simulink model "gm_test_phase_voltages_without_delays"  (R2022a)
settings: Solver=FixedStepDiscrete  StartTime=0.0  StopTime=10.0  RelTol=1e-3
undefined symbols (not defined in the file or in its folder): f_c, u_dc
libraries: hdlmdlgenlib x22, simulink x2
(part 2 of 5)

== system gm_test_phase_voltages_without_delays/Phase_voltages_per_switching_state1/Detect Rise Positive1/Positive ==
  u : Inport  OutDataTypeStr=boolean  SampleTime=1e-08
  Compare : RelationalOperator  Operator=>  OutDataTypeStr=boolean  ZeroCross=off
  Constant : Constant  DisableCoverage=on  Value=0  OutDataTypeStr=Inherit: Inherit via back propagation  SampleTime=-1  PreserveConstantTs=on
  y : Outport  SampleTime=1e-08
  wires:
  Compare/1 -> y/1
  Constant/1 -> Compare/2
  u/1 -> Compare/1

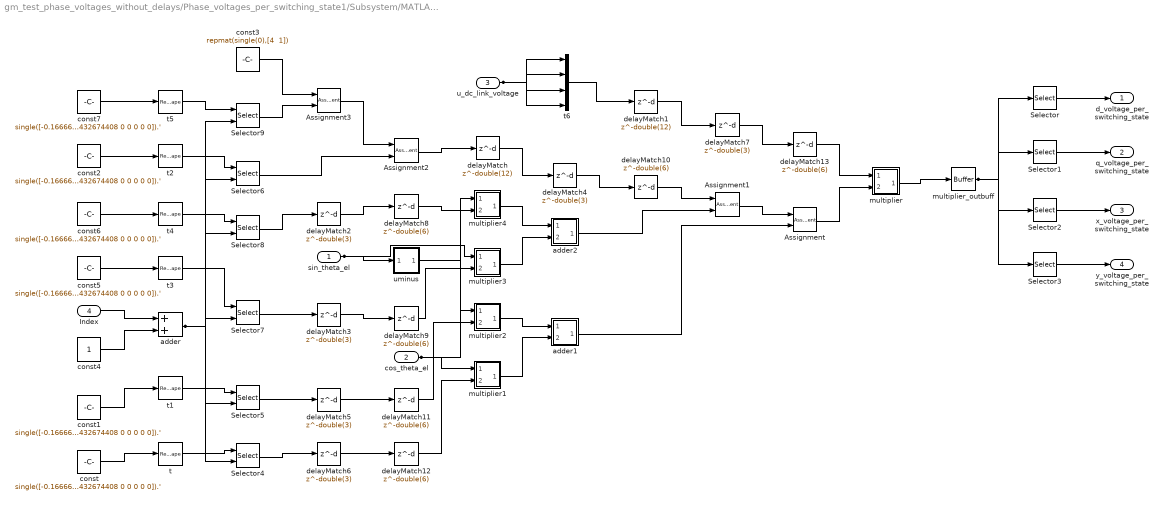
== system gm_test_phase_voltages_without_delays/Phase_voltages_per_switching_state1/Subsystem/MATLAB Function ==
  sin_theta_el : Inport  OutDataTypeStr=single  PortDimensions=1  SampleTime=1e-08
  cos_theta_el : Inport  Port=2  OutDataTypeStr=single  PortDimensions=1  SampleTime=1e-08
  u_dc_link_voltage : Inport  Port=3  OutDataTypeStr=single  PortDimensions=1  SampleTime=1e-08
  Index : Inport  Port=4  OutDataTypeStr=int32  PortDimensions=1  SampleTime=1e-08
  Assignment : Assignment  NumberOfDimensions=2  SampleTime=1e-08  IndexOptions=Index vector (dialog),Index vector (dialog)  Indices=double(2),double(1)  OutputSizes=double(0),double(0)
  Assignment1 : Assignment  NumberOfDimensions=2  SampleTime=1e-08  IndexOptions=Index vector (dialog),Index vector (dialog)  Indices=double(1),double(1)  OutputSizes=double(0),double(0)
  Assignment2 : Assignment  NumberOfDimensions=2  SampleTime=1e-08  IndexOptions=Index vector (dialog),Index vector (dialog)  Indices=double(4),double(1)  OutputSizes=double(0),double(0)
  Assignment3 : Assignment  NumberOfDimensions=2  SampleTime=1e-08  IndexOptions=Index vector (dialog),Index vector (dialog)  Indices=double(3),double(1)  OutputSizes=double(0),double(0)
  Selector : Selector  NumberOfDimensions=2  SampleTime=1e-08  IndexOptions=Index vector (dialog),Index vector (dialog)  Indices=double(1),double(1)  OutputSizes=double(0),double(0)
  Selector1 : Selector  NumberOfDimensions=2  SampleTime=1e-08  IndexOptions=Index vector (dialog),Index vector (dialog)  Indices=double(2),double(1)  OutputSizes=double(0),double(0)
  Selector2 : Selector  NumberOfDimensions=2  SampleTime=1e-08  IndexOptions=Index vector (dialog),Index vector (dialog)  Indices=double(3),double(1)  OutputSizes=double(0),double(0)
  Selector3 : Selector  NumberOfDimensions=2  SampleTime=1e-08  IndexOptions=Index vector (dialog),Index vector (dialog)  Indices=double(4),double(1)  OutputSizes=double(0),double(0)
  Selector4 : Selector  NumberOfDimensions=2  SampleTime=1e-08  IndexOptions=Index vector (dialog),Index vector (port)  Indices=double(2),double(-1)  OutputSizes=double(0),double(0)
  Selector5 : Selector  NumberOfDimensions=2  SampleTime=1e-08  IndexOptions=Index vector (dialog),Index vector (port)  Indices=double(1),double(-1)  OutputSizes=double(0),double(0)
  Selector6 : Selector  NumberOfDimensions=2  SampleTime=1e-08  IndexOptions=Index vector (dialog),Index vector (port)  Indices=double(4),double(-1)  OutputSizes=double(0),double(0)
  Selector7 : Selector  NumberOfDimensions=2  SampleTime=1e-08  IndexOptions=Index vector (dialog),Index vector (port)  Indices=double(2),double(-1)  OutputSizes=double(0),double(0)
  Selector8 : Selector  NumberOfDimensions=2  SampleTime=1e-08  IndexOptions=Index vector (dialog),Index vector (port)  Indices=double(1),double(-1)  OutputSizes=double(0),double(0)
  Selector9 : Selector  NumberOfDimensions=2  SampleTime=1e-08  IndexOptions=Index vector (dialog),Index vector (port)  Indices=double(3),double(-1)  OutputSizes=double(0),double(0)
  adder : Sum  AccumDataTypeStr=int32  OutDataTypeStr=int32  RndMeth=Nearest  SaturateOnIntegerOverflow=on  SampleTime=1e-08
  adder1 : Subsystem
      mask Display: disp('NFP\nadd');
  adder2 : Subsystem
      mask Display: disp('NFP\nadd');
  const{,1..2,5..7} (6 alike) : Constant  Value=single([-0.1666666716337204 -0.28867512941360474 -0.1666666716337204 0.28867512941360474 0.1666666716337204 -0.28867512941360474 0.1666666716337204 0.28867512941360474 -0.3333333432674408 0 -0.3333333432674408 0 0 0 0 0]).'  VectorParams1D=off  OutDataTypeStr=single  SampleTime=1e-08
  const3 : Constant  Value="repmat(single(0),[4  1])"  VectorParams1D=off  OutDataTypeStr=single  SampleTime=1e-08
  const4 : Constant  VectorParams1D=off  OutDataTypeStr=int32  SampleTime=1e-08
  delayMatch : Delay  DelayLength=double(12)  InitialCondition=0  SampleTime=1e-08
  delayMatch1 : Delay  DelayLength=double(12)  InitialCondition=0  SampleTime=1e-08
  delayMatch{8..13} (6 alike) : Delay  DelayLength=double(6)  InitialCondition=0  SampleTime=1e-08
  delayMatch{2..7} (6 alike) : Delay  DelayLength=double(3)  InitialCondition=0  SampleTime=1e-08
  multiplier : Subsystem
      mask Display: disp('NFP\nmul');
  multiplier1 : Subsystem
      mask Display: disp('NFP\nmul');
  multiplier2 : Subsystem
      mask Display: disp('NFP\nmul');
  multiplier3 : Subsystem
      mask Display: disp('NFP\nmul');
  multiplier4 : Subsystem
      mask Display: disp('NFP\nmul');
  multiplier_outbuff : hdlmdlgenlib/Buffer
      settings: SourceProductBaseCode=SL
  t{,1..5} (6 alike) : Reshape  OutputDimensionality=Customize  OutputDimensions=[4,4]
  t6 : Mux
  uminus : Subsystem
      mask Display: disp('NFP\numinus');
  d_voltage_per_switching_state : Outport  SampleTime=1e-08  VectorParamsAs1DForOutWhenUnconnected=off
  q_voltage_per_switching_state : Outport  Port=2  SampleTime=1e-08
  x_voltage_per_switching_state : Outport  Port=3  SampleTime=1e-08
  y_voltage_per_switching_state : Outport  Port=4  SampleTime=1e-08
  wires:
  Selector/1 -> d_voltage_per_switching_state/1
  Selector1/1 -> q_voltage_per_switching_state/1
  Selector2/1 -> x_voltage_per_switching_state/1
  Selector3/1 -> y_voltage_per_switching_state/1
  multiplier_outbuff/1 -> Selector3/1, Selector2/1, Selector1/1, Selector/1
  Assignment/1 -> multiplier/2(In2)
  Assignment1/1 -> Assignment/1
  delayMatch10/1 -> Assignment1/1
  delayMatch12/1 -> multiplier1/2(In2)
  delayMatch11/1 -> multiplier2/2(In2)
  Selector6/1 -> Assignment2/2
  Assignment3/1 -> Assignment2/1
  adder/1 -> Selector9/2, Selector8/2, Selector7/2, Selector6/2, Selector5/2, Selector4/2
  t/1 -> Selector4/1
  t1/1 -> Selector5/1
  delayMatch9/1 -> multiplier3/2(In2)
  delayMatch8/1 -> multiplier4/2(In2)
  t2/1 -> Selector6/1
  Selector9/1 -> Assignment3/2
  const3/1 -> Assignment3/1
  const4/1 -> adder/2
  t3/1 -> Selector7/1
  t4/1 -> Selector8/1
  t5/1 -> Selector9/1
  const/1 -> t/1
  const1/1 -> t1/1
  const2/1 -> t2/1
  const5/1 -> t3/1
  const6/1 -> t4/1
  const7/1 -> t5/1
  delayMatch13/1 -> multiplier/1(In1)
  multiplier/1(Out1) -> multiplier_outbuff/1
  adder1/1(Out1) -> Assignment/2
  multiplier1/1(Out1) -> adder1/2(In2)
  multiplier2/1(Out1) -> adder1/1(In1)
  adder2/1(Out1) -> Assignment1/2
  uminus/1(Out1) -> multiplier2/1(In1)
  multiplier3/1(Out1) -> adder2/2(In2)
  multiplier4/1(Out1) -> adder2/1(In1)
  Assignment2/1 -> delayMatch/1
  t6/1 -> delayMatch1/1
  Selector8/1 -> delayMatch2/1
  Selector7/1 -> delayMatch3/1
  delayMatch/1 -> delayMatch4/1
  Selector5/1 -> delayMatch5/1
  Selector4/1 -> delayMatch6/1
  delayMatch1/1 -> delayMatch7/1
  delayMatch2/1 -> delayMatch8/1
  delayMatch3/1 -> delayMatch9/1
  delayMatch4/1 -> delayMatch10/1
  delayMatch5/1 -> delayMatch11/1
  delayMatch6/1 -> delayMatch12/1
  delayMatch7/1 -> delayMatch13/1
  sin_theta_el/1 -> multiplier3/1(In1), uminus/1(In1)
  cos_theta_el/1 -> multiplier4/1(In1), multiplier1/1(In1)
  u_dc_link_voltage/1 -> t6/4, t6/3, t6/2, t6/1
  Index/1 -> adder/1

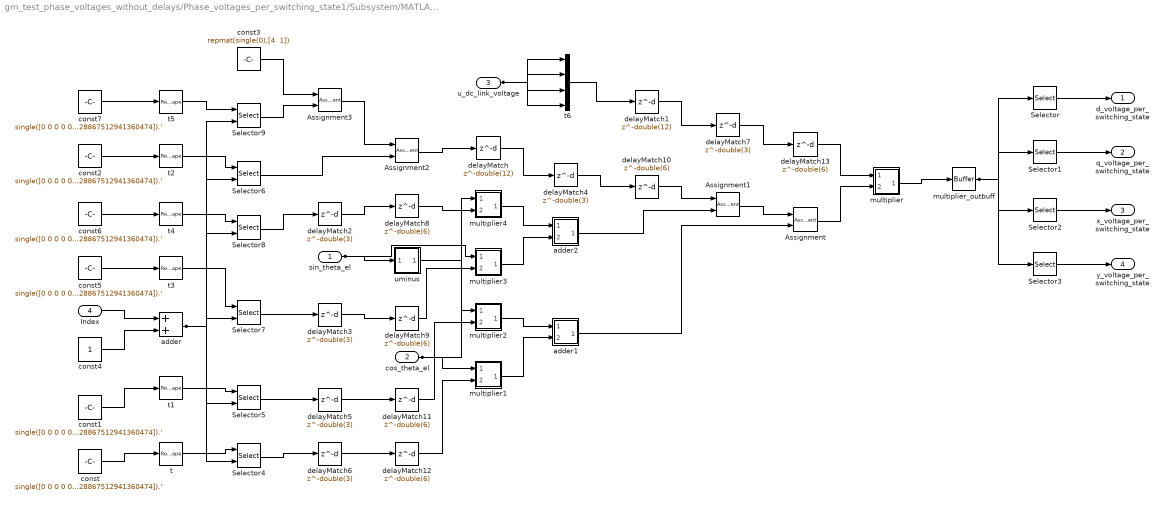
== system gm_test_phase_voltages_without_delays/Phase_voltages_per_switching_state1/Subsystem/MATLAB Function1 ==
  sin_theta_el : Inport  OutDataTypeStr=single  PortDimensions=1  SampleTime=1e-08
  cos_theta_el : Inport  Port=2  OutDataTypeStr=single  PortDimensions=1  SampleTime=1e-08
  u_dc_link_voltage : Inport  Port=3  OutDataTypeStr=single  PortDimensions=1  SampleTime=1e-08
  Index : Inport  Port=4  OutDataTypeStr=int32  PortDimensions=1  SampleTime=1e-08
  Assignment : Assignment  NumberOfDimensions=2  SampleTime=1e-08  IndexOptions=Index vector (dialog),Index vector (dialog)  Indices=double(2),double(1)  OutputSizes=double(0),double(0)
  Assignment1 : Assignment  NumberOfDimensions=2  SampleTime=1e-08  IndexOptions=Index vector (dialog),Index vector (dialog)  Indices=double(1),double(1)  OutputSizes=double(0),double(0)
  Assignment2 : Assignment  NumberOfDimensions=2  SampleTime=1e-08  IndexOptions=Index vector (dialog),Index vector (dialog)  Indices=double(4),double(1)  OutputSizes=double(0),double(0)
  Assignment3 : Assignment  NumberOfDimensions=2  SampleTime=1e-08  IndexOptions=Index vector (dialog),Index vector (dialog)  Indices=double(3),double(1)  OutputSizes=double(0),double(0)
  Selector : Selector  NumberOfDimensions=2  SampleTime=1e-08  IndexOptions=Index vector (dialog),Index vector (dialog)  Indices=double(1),double(1)  OutputSizes=double(0),double(0)
  Selector1 : Selector  NumberOfDimensions=2  SampleTime=1e-08  IndexOptions=Index vector (dialog),Index vector (dialog)  Indices=double(2),double(1)  OutputSizes=double(0),double(0)
  Selector2 : Selector  NumberOfDimensions=2  SampleTime=1e-08  IndexOptions=Index vector (dialog),Index vector (dialog)  Indices=double(3),double(1)  OutputSizes=double(0),double(0)
  Selector3 : Selector  NumberOfDimensions=2  SampleTime=1e-08  IndexOptions=Index vector (dialog),Index vector (dialog)  Indices=double(4),double(1)  OutputSizes=double(0),double(0)
  Selector4 : Selector  NumberOfDimensions=2  SampleTime=1e-08  IndexOptions=Index vector (dialog),Index vector (port)  Indices=double(2),double(-1)  OutputSizes=double(0),double(0)
  Selector5 : Selector  NumberOfDimensions=2  SampleTime=1e-08  IndexOptions=Index vector (dialog),Index vector (port)  Indices=double(1),double(-1)  OutputSizes=double(0),double(0)
  Selector6 : Selector  NumberOfDimensions=2  SampleTime=1e-08  IndexOptions=Index vector (dialog),Index vector (port)  Indices=double(4),double(-1)  OutputSizes=double(0),double(0)
  Selector7 : Selector  NumberOfDimensions=2  SampleTime=1e-08  IndexOptions=Index vector (dialog),Index vector (port)  Indices=double(2),double(-1)  OutputSizes=double(0),double(0)
  Selector8 : Selector  NumberOfDimensions=2  SampleTime=1e-08  IndexOptions=Index vector (dialog),Index vector (port)  Indices=double(1),double(-1)  OutputSizes=double(0),double(0)
  Selector9 : Selector  NumberOfDimensions=2  SampleTime=1e-08  IndexOptions=Index vector (dialog),Index vector (port)  Indices=double(3),double(-1)  OutputSizes=double(0),double(0)
  adder : Sum  AccumDataTypeStr=int32  OutDataTypeStr=int32  RndMeth=Nearest  SaturateOnIntegerOverflow=on  SampleTime=1e-08
  adder1 : Subsystem
      mask Display: disp('NFP\nadd');
  adder2 : Subsystem
      mask Display: disp('NFP\nadd');
  const{,1..2,5..7} (6 alike) : Constant  Value=single([0 0 0 0 0.3333333432674408 0 0.3333333432674408 0 -0.1666666716337204 0.28867512941360474 -0.1666666716337204 -0.28867512941360474 0.1666666716337204 0.28867512941360474 0.1666666716337204 -0.28867512941360474]).'  VectorParams1D=off  OutDataTypeStr=single  SampleTime=1e-08
  const3 : Constant  Value="repmat(single(0),[4  1])"  VectorParams1D=off  OutDataTypeStr=single  SampleTime=1e-08
  const4 : Constant  VectorParams1D=off  OutDataTypeStr=int32  SampleTime=1e-08
  delayMatch : Delay  DelayLength=double(12)  InitialCondition=0  SampleTime=1e-08
  delayMatch1 : Delay  DelayLength=double(12)  InitialCondition=0  SampleTime=1e-08
  delayMatch{8..13} (6 alike) : Delay  DelayLength=double(6)  InitialCondition=0  SampleTime=1e-08
  delayMatch{2..7} (6 alike) : Delay  DelayLength=double(3)  InitialCondition=0  SampleTime=1e-08
  multiplier : Subsystem
      mask Display: disp('NFP\nmul');
  multiplier1 : Subsystem
      mask Display: disp('NFP\nmul');
  multiplier2 : Subsystem
      mask Display: disp('NFP\nmul');
  multiplier3 : Subsystem
      mask Display: disp('NFP\nmul');
  multiplier4 : Subsystem
      mask Display: disp('NFP\nmul');
  multiplier_outbuff : hdlmdlgenlib/Buffer
      settings: SourceProductBaseCode=SL
  t{,1..5} (6 alike) : Reshape  OutputDimensionality=Customize  OutputDimensions=[4,4]
  t6 : Mux
  uminus : Subsystem
      mask Display: disp('NFP\numinus');
  d_voltage_per_switching_state : Outport  SampleTime=1e-08  VectorParamsAs1DForOutWhenUnconnected=off
  q_voltage_per_switching_state : Outport  Port=2  SampleTime=1e-08
  x_voltage_per_switching_state : Outport  Port=3  SampleTime=1e-08
  y_voltage_per_switching_state : Outport  Port=4  SampleTime=1e-08
  wires:
  Selector/1 -> d_voltage_per_switching_state/1
  Selector1/1 -> q_voltage_per_switching_state/1
  Selector2/1 -> x_voltage_per_switching_state/1
  Selector3/1 -> y_voltage_per_switching_state/1
  multiplier_outbuff/1 -> Selector3/1, Selector2/1, Selector1/1, Selector/1
  Assignment/1 -> multiplier/2(In2)
  Assignment1/1 -> Assignment/1
  delayMatch10/1 -> Assignment1/1
  delayMatch12/1 -> multiplier1/2(In2)
  delayMatch11/1 -> multiplier2/2(In2)
  Selector6/1 -> Assignment2/2
  Assignment3/1 -> Assignment2/1
  adder/1 -> Selector9/2, Selector8/2, Selector7/2, Selector6/2, Selector5/2, Selector4/2
  t/1 -> Selector4/1
  t1/1 -> Selector5/1
  delayMatch9/1 -> multiplier3/2(In2)
  delayMatch8/1 -> multiplier4/2(In2)
  t2/1 -> Selector6/1
  Selector9/1 -> Assignment3/2
  const3/1 -> Assignment3/1
  const4/1 -> adder/2
  t3/1 -> Selector7/1
  t4/1 -> Selector8/1
  t5/1 -> Selector9/1
  const/1 -> t/1
  const1/1 -> t1/1
  const2/1 -> t2/1
  const5/1 -> t3/1
  const6/1 -> t4/1
  const7/1 -> t5/1
  delayMatch13/1 -> multiplier/1(In1)
  multiplier/1(Out1) -> multiplier_outbuff/1
  adder1/1(Out1) -> Assignment/2
  multiplier1/1(Out1) -> adder1/2(In2)
  multiplier2/1(Out1) -> adder1/1(In1)
  adder2/1(Out1) -> Assignment1/2
  uminus/1(Out1) -> multiplier2/1(In1)
  multiplier3/1(Out1) -> adder2/2(In2)
  multiplier4/1(Out1) -> adder2/1(In1)
  Assignment2/1 -> delayMatch/1
  t6/1 -> delayMatch1/1
  Selector8/1 -> delayMatch2/1
  Selector7/1 -> delayMatch3/1
  delayMatch/1 -> delayMatch4/1
  Selector5/1 -> delayMatch5/1
  Selector4/1 -> delayMatch6/1
  delayMatch1/1 -> delayMatch7/1
  delayMatch2/1 -> delayMatch8/1
  delayMatch3/1 -> delayMatch9/1
  delayMatch4/1 -> delayMatch10/1
  delayMatch5/1 -> delayMatch11/1
  delayMatch6/1 -> delayMatch12/1
  delayMatch7/1 -> delayMatch13/1
  sin_theta_el/1 -> multiplier3/1(In1), uminus/1(In1)
  cos_theta_el/1 -> multiplier4/1(In1), multiplier1/1(In1)
  u_dc_link_voltage/1 -> t6/4, t6/3, t6/2, t6/1
  Index/1 -> adder/1

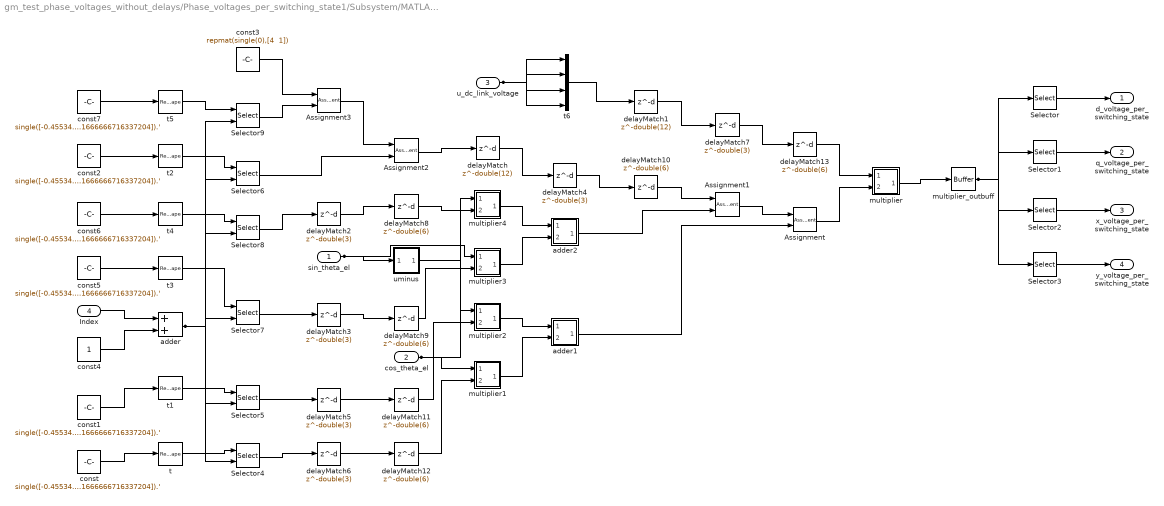
== system gm_test_phase_voltages_without_delays/Phase_voltages_per_switching_state1/Subsystem/MATLAB Function10 ==
  sin_theta_el : Inport  OutDataTypeStr=single  PortDimensions=1  SampleTime=1e-08
  cos_theta_el : Inport  Port=2  OutDataTypeStr=single  PortDimensions=1  SampleTime=1e-08
  u_dc_link_voltage : Inport  Port=3  OutDataTypeStr=single  PortDimensions=1  SampleTime=1e-08
  Index : Inport  Port=4  OutDataTypeStr=int32  PortDimensions=1  SampleTime=1e-08
  Assignment : Assignment  NumberOfDimensions=2  SampleTime=1e-08  IndexOptions=Index vector (dialog),Index vector (dialog)  Indices=double(2),double(1)  OutputSizes=double(0),double(0)
  Assignment1 : Assignment  NumberOfDimensions=2  SampleTime=1e-08  IndexOptions=Index vector (dialog),Index vector (dialog)  Indices=double(1),double(1)  OutputSizes=double(0),double(0)
  Assignment2 : Assignment  NumberOfDimensions=2  SampleTime=1e-08  IndexOptions=Index vector (dialog),Index vector (dialog)  Indices=double(4),double(1)  OutputSizes=double(0),double(0)
  Assignment3 : Assignment  NumberOfDimensions=2  SampleTime=1e-08  IndexOptions=Index vector (dialog),Index vector (dialog)  Indices=double(3),double(1)  OutputSizes=double(0),double(0)
  Selector : Selector  NumberOfDimensions=2  SampleTime=1e-08  IndexOptions=Index vector (dialog),Index vector (dialog)  Indices=double(1),double(1)  OutputSizes=double(0),double(0)
  Selector1 : Selector  NumberOfDimensions=2  SampleTime=1e-08  IndexOptions=Index vector (dialog),Index vector (dialog)  Indices=double(2),double(1)  OutputSizes=double(0),double(0)
  Selector2 : Selector  NumberOfDimensions=2  SampleTime=1e-08  IndexOptions=Index vector (dialog),Index vector (dialog)  Indices=double(3),double(1)  OutputSizes=double(0),double(0)
  Selector3 : Selector  NumberOfDimensions=2  SampleTime=1e-08  IndexOptions=Index vector (dialog),Index vector (dialog)  Indices=double(4),double(1)  OutputSizes=double(0),double(0)
  Selector4 : Selector  NumberOfDimensions=2  SampleTime=1e-08  IndexOptions=Index vector (dialog),Index vector (port)  Indices=double(2),double(-1)  OutputSizes=double(0),double(0)
  Selector5 : Selector  NumberOfDimensions=2  SampleTime=1e-08  IndexOptions=Index vector (dialog),Index vector (port)  Indices=double(1),double(-1)  OutputSizes=double(0),double(0)
  Selector6 : Selector  NumberOfDimensions=2  SampleTime=1e-08  IndexOptions=Index vector (dialog),Index vector (port)  Indices=double(4),double(-1)  OutputSizes=double(0),double(0)
  Selector7 : Selector  NumberOfDimensions=2  SampleTime=1e-08  IndexOptions=Index vector (dialog),Index vector (port)  Indices=double(2),double(-1)  OutputSizes=double(0),double(0)
  Selector8 : Selector  NumberOfDimensions=2  SampleTime=1e-08  IndexOptions=Index vector (dialog),Index vector (port)  Indices=double(1),double(-1)  OutputSizes=double(0),double(0)
  Selector9 : Selector  NumberOfDimensions=2  SampleTime=1e-08  IndexOptions=Index vector (dialog),Index vector (port)  Indices=double(3),double(-1)  OutputSizes=double(0),double(0)
  adder : Sum  AccumDataTypeStr=int32  OutDataTypeStr=int32  RndMeth=Nearest  SaturateOnIntegerOverflow=on  SampleTime=1e-08
  adder1 : Subsystem
      mask Display: disp('NFP\nadd');
  adder2 : Subsystem
      mask Display: disp('NFP\nadd');
  const{,1..2,5..7} (6 alike) : Constant  Value=single([-0.45534181594848633 -0.12200846523046494 0.12200846523046494 0.45534181594848633 -0.12200846523046494 -0.12200846523046494 0.45534181594848633 0.45534181594848633 -0.6220084428787231 0.1666666716337204 -0.044658198952674866 0.1666666716337204 -0.28867512941360474 0.1666666716337204 0.28867512941360474 0.1666666716337204]).'  VectorParams1D=off  OutDataTypeStr=single  SampleTime=1e-08
  const3 : Constant  Value="repmat(single(0),[4  1])"  VectorParams1D=off  OutDataTypeStr=single  SampleTime=1e-08
  const4 : Constant  VectorParams1D=off  OutDataTypeStr=int32  SampleTime=1e-08
  delayMatch : Delay  DelayLength=double(12)  InitialCondition=0  SampleTime=1e-08
  delayMatch1 : Delay  DelayLength=double(12)  InitialCondition=0  SampleTime=1e-08
  delayMatch{8..13} (6 alike) : Delay  DelayLength=double(6)  InitialCondition=0  SampleTime=1e-08
  delayMatch{2..7} (6 alike) : Delay  DelayLength=double(3)  InitialCondition=0  SampleTime=1e-08
  multiplier : Subsystem
      mask Display: disp('NFP\nmul');
  multiplier1 : Subsystem
      mask Display: disp('NFP\nmul');
  multiplier2 : Subsystem
      mask Display: disp('NFP\nmul');
  multiplier3 : Subsystem
      mask Display: disp('NFP\nmul');
  multiplier4 : Subsystem
      mask Display: disp('NFP\nmul');
  multiplier_outbuff : hdlmdlgenlib/Buffer
      settings: SourceProductBaseCode=SL
  t{,1..5} (6 alike) : Reshape  OutputDimensionality=Customize  OutputDimensions=[4,4]
  t6 : Mux
  uminus : Subsystem
      mask Display: disp('NFP\numinus');
  d_voltage_per_switching_state : Outport  SampleTime=1e-08  VectorParamsAs1DForOutWhenUnconnected=off
  q_voltage_per_switching_state : Outport  Port=2  SampleTime=1e-08
  x_voltage_per_switching_state : Outport  Port=3  SampleTime=1e-08
  y_voltage_per_switching_state : Outport  Port=4  SampleTime=1e-08
  wires:
  Selector/1 -> d_voltage_per_switching_state/1
  Selector1/1 -> q_voltage_per_switching_state/1
  Selector2/1 -> x_voltage_per_switching_state/1
  Selector3/1 -> y_voltage_per_switching_state/1
  multiplier_outbuff/1 -> Selector3/1, Selector2/1, Selector1/1, Selector/1
  Assignment/1 -> multiplier/2(In2)
  Assignment1/1 -> Assignment/1
  delayMatch10/1 -> Assignment1/1
  delayMatch12/1 -> multiplier1/2(In2)
  delayMatch11/1 -> multiplier2/2(In2)
  Selector6/1 -> Assignment2/2
  Assignment3/1 -> Assignment2/1
  adder/1 -> Selector9/2, Selector8/2, Selector7/2, Selector6/2, Selector5/2, Selector4/2
  t/1 -> Selector4/1
  t1/1 -> Selector5/1
  delayMatch9/1 -> multiplier3/2(In2)
  delayMatch8/1 -> multiplier4/2(In2)
  t2/1 -> Selector6/1
  Selector9/1 -> Assignment3/2
  const3/1 -> Assignment3/1
  const4/1 -> adder/2
  t3/1 -> Selector7/1
  t4/1 -> Selector8/1
  t5/1 -> Selector9/1
  const/1 -> t/1
  const1/1 -> t1/1
  const2/1 -> t2/1
  const5/1 -> t3/1
  const6/1 -> t4/1
  const7/1 -> t5/1
  delayMatch13/1 -> multiplier/1(In1)
  multiplier/1(Out1) -> multiplier_outbuff/1
  adder1/1(Out1) -> Assignment/2
  multiplier1/1(Out1) -> adder1/2(In2)
  multiplier2/1(Out1) -> adder1/1(In1)
  adder2/1(Out1) -> Assignment1/2
  uminus/1(Out1) -> multiplier2/1(In1)
  multiplier3/1(Out1) -> adder2/2(In2)
  multiplier4/1(Out1) -> adder2/1(In1)
  Assignment2/1 -> delayMatch/1
  t6/1 -> delayMatch1/1
  Selector8/1 -> delayMatch2/1
  Selector7/1 -> delayMatch3/1
  delayMatch/1 -> delayMatch4/1
  Selector5/1 -> delayMatch5/1
  Selector4/1 -> delayMatch6/1
  delayMatch1/1 -> delayMatch7/1
  delayMatch2/1 -> delayMatch8/1
  delayMatch3/1 -> delayMatch9/1
  delayMatch4/1 -> delayMatch10/1
  delayMatch5/1 -> delayMatch11/1
  delayMatch6/1 -> delayMatch12/1
  delayMatch7/1 -> delayMatch13/1
  sin_theta_el/1 -> multiplier3/1(In1), uminus/1(In1)
  cos_theta_el/1 -> multiplier4/1(In1), multiplier1/1(In1)
  u_dc_link_voltage/1 -> t6/4, t6/3, t6/2, t6/1
  Index/1 -> adder/1

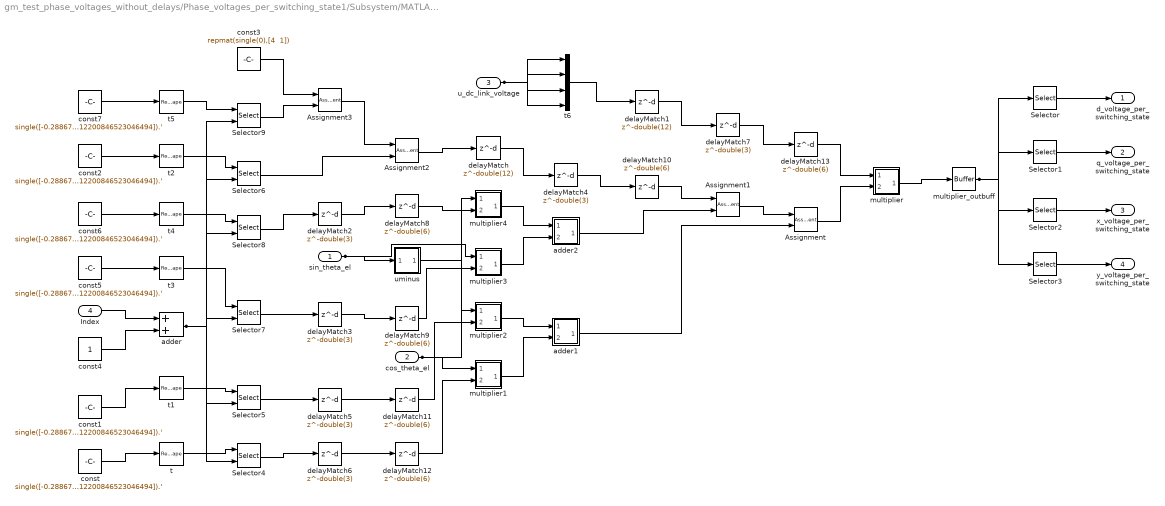
== system gm_test_phase_voltages_without_delays/Phase_voltages_per_switching_state1/Subsystem/MATLAB Function11 ==
  sin_theta_el : Inport  OutDataTypeStr=single  PortDimensions=1  SampleTime=1e-08
  cos_theta_el : Inport  Port=2  OutDataTypeStr=single  PortDimensions=1  SampleTime=1e-08
  u_dc_link_voltage : Inport  Port=3  OutDataTypeStr=single  PortDimensions=1  SampleTime=1e-08
  Index : Inport  Port=4  OutDataTypeStr=int32  PortDimensions=1  SampleTime=1e-08
  Assignment : Assignment  NumberOfDimensions=2  SampleTime=1e-08  IndexOptions=Index vector (dialog),Index vector (dialog)  Indices=double(2),double(1)  OutputSizes=double(0),double(0)
  Assignment1 : Assignment  NumberOfDimensions=2  SampleTime=1e-08  IndexOptions=Index vector (dialog),Index vector (dialog)  Indices=double(1),double(1)  OutputSizes=double(0),double(0)
  Assignment2 : Assignment  NumberOfDimensions=2  SampleTime=1e-08  IndexOptions=Index vector (dialog),Index vector (dialog)  Indices=double(4),double(1)  OutputSizes=double(0),double(0)
  Assignment3 : Assignment  NumberOfDimensions=2  SampleTime=1e-08  IndexOptions=Index vector (dialog),Index vector (dialog)  Indices=double(3),double(1)  OutputSizes=double(0),double(0)
  Selector : Selector  NumberOfDimensions=2  SampleTime=1e-08  IndexOptions=Index vector (dialog),Index vector (dialog)  Indices=double(1),double(1)  OutputSizes=double(0),double(0)
  Selector1 : Selector  NumberOfDimensions=2  SampleTime=1e-08  IndexOptions=Index vector (dialog),Index vector (dialog)  Indices=double(2),double(1)  OutputSizes=double(0),double(0)
  Selector2 : Selector  NumberOfDimensions=2  SampleTime=1e-08  IndexOptions=Index vector (dialog),Index vector (dialog)  Indices=double(3),double(1)  OutputSizes=double(0),double(0)
  Selector3 : Selector  NumberOfDimensions=2  SampleTime=1e-08  IndexOptions=Index vector (dialog),Index vector (dialog)  Indices=double(4),double(1)  OutputSizes=double(0),double(0)
  Selector4 : Selector  NumberOfDimensions=2  SampleTime=1e-08  IndexOptions=Index vector (dialog),Index vector (port)  Indices=double(2),double(-1)  OutputSizes=double(0),double(0)
  Selector5 : Selector  NumberOfDimensions=2  SampleTime=1e-08  IndexOptions=Index vector (dialog),Index vector (port)  Indices=double(1),double(-1)  OutputSizes=double(0),double(0)
  Selector6 : Selector  NumberOfDimensions=2  SampleTime=1e-08  IndexOptions=Index vector (dialog),Index vector (port)  Indices=double(4),double(-1)  OutputSizes=double(0),double(0)
  Selector7 : Selector  NumberOfDimensions=2  SampleTime=1e-08  IndexOptions=Index vector (dialog),Index vector (port)  Indices=double(2),double(-1)  OutputSizes=double(0),double(0)
  Selector8 : Selector  NumberOfDimensions=2  SampleTime=1e-08  IndexOptions=Index vector (dialog),Index vector (port)  Indices=double(1),double(-1)  OutputSizes=double(0),double(0)
  Selector9 : Selector  NumberOfDimensions=2  SampleTime=1e-08  IndexOptions=Index vector (dialog),Index vector (port)  Indices=double(3),double(-1)  OutputSizes=double(0),double(0)
  adder : Sum  AccumDataTypeStr=int32  OutDataTypeStr=int32  RndMeth=Nearest  SaturateOnIntegerOverflow=on  SampleTime=1e-08
  adder1 : Subsystem
      mask Display: disp('NFP\nadd');
  adder2 : Subsystem
      mask Display: disp('NFP\nadd');
  const{,1..2,5..7} (6 alike) : Constant  Value=single([-0.28867512941360474 0.1666666716337204 0.28867512941360474 0.1666666716337204 0.044658198952674866 0.1666666716337204 0.6220084428787231 0.1666666716337204 -0.45534181594848633 0.45534181594848633 0.12200846523046494 -0.12200846523046494 -0.12200846523046494 0.45534181594848633 0.45534181594848633 -0.12200846523046494]).'  VectorParams1D=off  OutDataTypeStr=single  SampleTime=1e-08
  const3 : Constant  Value="repmat(single(0),[4  1])"  VectorParams1D=off  OutDataTypeStr=single  SampleTime=1e-08
  const4 : Constant  VectorParams1D=off  OutDataTypeStr=int32  SampleTime=1e-08
  delayMatch : Delay  DelayLength=double(12)  InitialCondition=0  SampleTime=1e-08
  delayMatch1 : Delay  DelayLength=double(12)  InitialCondition=0  SampleTime=1e-08
  delayMatch{8..13} (6 alike) : Delay  DelayLength=double(6)  InitialCondition=0  SampleTime=1e-08
  delayMatch{2..7} (6 alike) : Delay  DelayLength=double(3)  InitialCondition=0  SampleTime=1e-08
  multiplier : Subsystem
      mask Display: disp('NFP\nmul');
  multiplier1 : Subsystem
      mask Display: disp('NFP\nmul');
  multiplier2 : Subsystem
      mask Display: disp('NFP\nmul');
  multiplier3 : Subsystem
      mask Display: disp('NFP\nmul');
  multiplier4 : Subsystem
      mask Display: disp('NFP\nmul');
  multiplier_outbuff : hdlmdlgenlib/Buffer
      settings: SourceProductBaseCode=SL
  t{,1..5} (6 alike) : Reshape  OutputDimensionality=Customize  OutputDimensions=[4,4]
  t6 : Mux
  uminus : Subsystem
      mask Display: disp('NFP\numinus');
  d_voltage_per_switching_state : Outport  SampleTime=1e-08  VectorParamsAs1DForOutWhenUnconnected=off
  q_voltage_per_switching_state : Outport  Port=2  SampleTime=1e-08
  x_voltage_per_switching_state : Outport  Port=3  SampleTime=1e-08
  y_voltage_per_switching_state : Outport  Port=4  SampleTime=1e-08
  wires:
  Selector/1 -> d_voltage_per_switching_state/1
  Selector1/1 -> q_voltage_per_switching_state/1
  Selector2/1 -> x_voltage_per_switching_state/1
  Selector3/1 -> y_voltage_per_switching_state/1
  multiplier_outbuff/1 -> Selector3/1, Selector2/1, Selector1/1, Selector/1
  Assignment/1 -> multiplier/2(In2)
  Assignment1/1 -> Assignment/1
  delayMatch10/1 -> Assignment1/1
  delayMatch12/1 -> multiplier1/2(In2)
  delayMatch11/1 -> multiplier2/2(In2)
  Selector6/1 -> Assignment2/2
  Assignment3/1 -> Assignment2/1
  adder/1 -> Selector9/2, Selector8/2, Selector7/2, Selector6/2, Selector5/2, Selector4/2
  t/1 -> Selector4/1
  t1/1 -> Selector5/1
  delayMatch9/1 -> multiplier3/2(In2)
  delayMatch8/1 -> multiplier4/2(In2)
  t2/1 -> Selector6/1
  Selector9/1 -> Assignment3/2
  const3/1 -> Assignment3/1
  const4/1 -> adder/2
  t3/1 -> Selector7/1
  t4/1 -> Selector8/1
  t5/1 -> Selector9/1
  const/1 -> t/1
  const1/1 -> t1/1
  const2/1 -> t2/1
  const5/1 -> t3/1
  const6/1 -> t4/1
  const7/1 -> t5/1
  delayMatch13/1 -> multiplier/1(In1)
  multiplier/1(Out1) -> multiplier_outbuff/1
  adder1/1(Out1) -> Assignment/2
  multiplier1/1(Out1) -> adder1/2(In2)
  multiplier2/1(Out1) -> adder1/1(In1)
  adder2/1(Out1) -> Assignment1/2
  uminus/1(Out1) -> multiplier2/1(In1)
  multiplier3/1(Out1) -> adder2/2(In2)
  multiplier4/1(Out1) -> adder2/1(In1)
  Assignment2/1 -> delayMatch/1
  t6/1 -> delayMatch1/1
  Selector8/1 -> delayMatch2/1
  Selector7/1 -> delayMatch3/1
  delayMatch/1 -> delayMatch4/1
  Selector5/1 -> delayMatch5/1
  Selector4/1 -> delayMatch6/1
  delayMatch1/1 -> delayMatch7/1
  delayMatch2/1 -> delayMatch8/1
  delayMatch3/1 -> delayMatch9/1
  delayMatch4/1 -> delayMatch10/1
  delayMatch5/1 -> delayMatch11/1
  delayMatch6/1 -> delayMatch12/1
  delayMatch7/1 -> delayMatch13/1
  sin_theta_el/1 -> multiplier3/1(In1), uminus/1(In1)
  cos_theta_el/1 -> multiplier4/1(In1), multiplier1/1(In1)
  u_dc_link_voltage/1 -> t6/4, t6/3, t6/2, t6/1
  Index/1 -> adder/1

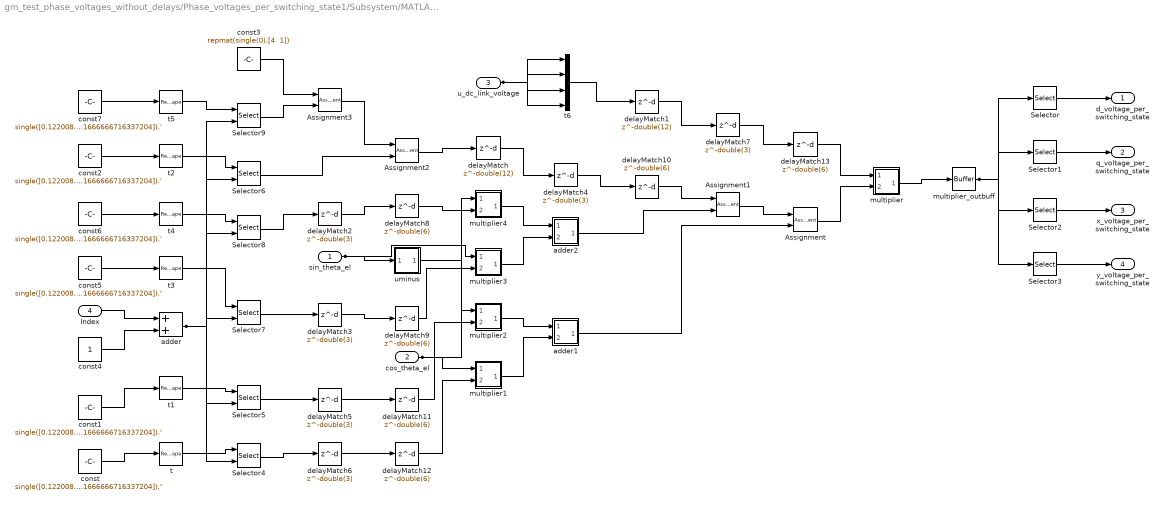
== system gm_test_phase_voltages_without_delays/Phase_voltages_per_switching_state1/Subsystem/MATLAB Function12 ==
  sin_theta_el : Inport  OutDataTypeStr=single  PortDimensions=1  SampleTime=1e-08
  cos_theta_el : Inport  Port=2  OutDataTypeStr=single  PortDimensions=1  SampleTime=1e-08
  u_dc_link_voltage : Inport  Port=3  OutDataTypeStr=single  PortDimensions=1  SampleTime=1e-08
  Index : Inport  Port=4  OutDataTypeStr=int32  PortDimensions=1  SampleTime=1e-08
  Assignment : Assignment  NumberOfDimensions=2  SampleTime=1e-08  IndexOptions=Index vector (dialog),Index vector (dialog)  Indices=double(2),double(1)  OutputSizes=double(0),double(0)
  Assignment1 : Assignment  NumberOfDimensions=2  SampleTime=1e-08  IndexOptions=Index vector (dialog),Index vector (dialog)  Indices=double(1),double(1)  OutputSizes=double(0),double(0)
  Assignment2 : Assignment  NumberOfDimensions=2  SampleTime=1e-08  IndexOptions=Index vector (dialog),Index vector (dialog)  Indices=double(4),double(1)  OutputSizes=double(0),double(0)
  Assignment3 : Assignment  NumberOfDimensions=2  SampleTime=1e-08  IndexOptions=Index vector (dialog),Index vector (dialog)  Indices=double(3),double(1)  OutputSizes=double(0),double(0)
  Selector : Selector  NumberOfDimensions=2  SampleTime=1e-08  IndexOptions=Index vector (dialog),Index vector (dialog)  Indices=double(1),double(1)  OutputSizes=double(0),double(0)
  Selector1 : Selector  NumberOfDimensions=2  SampleTime=1e-08  IndexOptions=Index vector (dialog),Index vector (dialog)  Indices=double(2),double(1)  OutputSizes=double(0),double(0)
  Selector2 : Selector  NumberOfDimensions=2  SampleTime=1e-08  IndexOptions=Index vector (dialog),Index vector (dialog)  Indices=double(3),double(1)  OutputSizes=double(0),double(0)
  Selector3 : Selector  NumberOfDimensions=2  SampleTime=1e-08  IndexOptions=Index vector (dialog),Index vector (dialog)  Indices=double(4),double(1)  OutputSizes=double(0),double(0)
  Selector4 : Selector  NumberOfDimensions=2  SampleTime=1e-08  IndexOptions=Index vector (dialog),Index vector (port)  Indices=double(2),double(-1)  OutputSizes=double(0),double(0)
  Selector5 : Selector  NumberOfDimensions=2  SampleTime=1e-08  IndexOptions=Index vector (dialog),Index vector (port)  Indices=double(1),double(-1)  OutputSizes=double(0),double(0)
  Selector6 : Selector  NumberOfDimensions=2  SampleTime=1e-08  IndexOptions=Index vector (dialog),Index vector (port)  Indices=double(4),double(-1)  OutputSizes=double(0),double(0)
  Selector7 : Selector  NumberOfDimensions=2  SampleTime=1e-08  IndexOptions=Index vector (dialog),Index vector (port)  Indices=double(2),double(-1)  OutputSizes=double(0),double(0)
  Selector8 : Selector  NumberOfDimensions=2  SampleTime=1e-08  IndexOptions=Index vector (dialog),Index vector (port)  Indices=double(1),double(-1)  OutputSizes=double(0),double(0)
  Selector9 : Selector  NumberOfDimensions=2  SampleTime=1e-08  IndexOptions=Index vector (dialog),Index vector (port)  Indices=double(3),double(-1)  OutputSizes=double(0),double(0)
  adder : Sum  AccumDataTypeStr=int32  OutDataTypeStr=int32  RndMeth=Nearest  SaturateOnIntegerOverflow=on  SampleTime=1e-08
  adder1 : Subsystem
      mask Display: disp('NFP\nadd');
  adder2 : Subsystem
      mask Display: disp('NFP\nadd');
  const{,1..2,5..7} (6 alike) : Constant  Value=single([0.12200846523046494 -0.12200846523046494 -0.45534181594848633 0.45534181594848633 0.45534181594848633 -0.12200846523046494 -0.12200846523046494 0.45534181594848633 -0.044658198952674866 0.1666666716337204 -0.6220084428787231 0.1666666716337204 0.28867512941360474 0.1666666716337204 -0.28867512941360474 0.1666666716337204]).'  VectorParams1D=off  OutDataTypeStr=single  SampleTime=1e-08
  const3 : Constant  Value="repmat(single(0),[4  1])"  VectorParams1D=off  OutDataTypeStr=single  SampleTime=1e-08
  const4 : Constant  VectorParams1D=off  OutDataTypeStr=int32  SampleTime=1e-08
  delayMatch : Delay  DelayLength=double(12)  InitialCondition=0  SampleTime=1e-08
  delayMatch1 : Delay  DelayLength=double(12)  InitialCondition=0  SampleTime=1e-08
  delayMatch{8..13} (6 alike) : Delay  DelayLength=double(6)  InitialCondition=0  SampleTime=1e-08
  delayMatch{2..7} (6 alike) : Delay  DelayLength=double(3)  InitialCondition=0  SampleTime=1e-08
  multiplier : Subsystem
      mask Display: disp('NFP\nmul');
  multiplier1 : Subsystem
      mask Display: disp('NFP\nmul');
  multiplier2 : Subsystem
      mask Display: disp('NFP\nmul');
  multiplier3 : Subsystem
      mask Display: disp('NFP\nmul');
  multiplier4 : Subsystem
      mask Display: disp('NFP\nmul');
  multiplier_outbuff : hdlmdlgenlib/Buffer
      settings: SourceProductBaseCode=SL
  t{,1..5} (6 alike) : Reshape  OutputDimensionality=Customize  OutputDimensions=[4,4]
  t6 : Mux
  uminus : Subsystem
      mask Display: disp('NFP\numinus');
  d_voltage_per_switching_state : Outport  SampleTime=1e-08  VectorParamsAs1DForOutWhenUnconnected=off
  q_voltage_per_switching_state : Outport  Port=2  SampleTime=1e-08
  x_voltage_per_switching_state : Outport  Port=3  SampleTime=1e-08
  y_voltage_per_switching_state : Outport  Port=4  SampleTime=1e-08
  wires:
  Selector/1 -> d_voltage_per_switching_state/1
  Selector1/1 -> q_voltage_per_switching_state/1
  Selector2/1 -> x_voltage_per_switching_state/1
  Selector3/1 -> y_voltage_per_switching_state/1
  multiplier_outbuff/1 -> Selector3/1, Selector2/1, Selector1/1, Selector/1
  Assignment/1 -> multiplier/2(In2)
  Assignment1/1 -> Assignment/1
  delayMatch10/1 -> Assignment1/1
  delayMatch12/1 -> multiplier1/2(In2)
  delayMatch11/1 -> multiplier2/2(In2)
  Selector6/1 -> Assignment2/2
  Assignment3/1 -> Assignment2/1
  adder/1 -> Selector9/2, Selector8/2, Selector7/2, Selector6/2, Selector5/2, Selector4/2
  t/1 -> Selector4/1
  t1/1 -> Selector5/1
  delayMatch9/1 -> multiplier3/2(In2)
  delayMatch8/1 -> multiplier4/2(In2)
  t2/1 -> Selector6/1
  Selector9/1 -> Assignment3/2
  const3/1 -> Assignment3/1
  const4/1 -> adder/2
  t3/1 -> Selector7/1
  t4/1 -> Selector8/1
  t5/1 -> Selector9/1
  const/1 -> t/1
  const1/1 -> t1/1
  const2/1 -> t2/1
  const5/1 -> t3/1
  const6/1 -> t4/1
  const7/1 -> t5/1
  delayMatch13/1 -> multiplier/1(In1)
  multiplier/1(Out1) -> multiplier_outbuff/1
  adder1/1(Out1) -> Assignment/2
  multiplier1/1(Out1) -> adder1/2(In2)
  multiplier2/1(Out1) -> adder1/1(In1)
  adder2/1(Out1) -> Assignment1/2
  uminus/1(Out1) -> multiplier2/1(In1)
  multiplier3/1(Out1) -> adder2/2(In2)
  multiplier4/1(Out1) -> adder2/1(In1)
  Assignment2/1 -> delayMatch/1
  t6/1 -> delayMatch1/1
  Selector8/1 -> delayMatch2/1
  Selector7/1 -> delayMatch3/1
  delayMatch/1 -> delayMatch4/1
  Selector5/1 -> delayMatch5/1
  Selector4/1 -> delayMatch6/1
  delayMatch1/1 -> delayMatch7/1
  delayMatch2/1 -> delayMatch8/1
  delayMatch3/1 -> delayMatch9/1
  delayMatch4/1 -> delayMatch10/1
  delayMatch5/1 -> delayMatch11/1
  delayMatch6/1 -> delayMatch12/1
  delayMatch7/1 -> delayMatch13/1
  sin_theta_el/1 -> multiplier3/1(In1), uminus/1(In1)
  cos_theta_el/1 -> multiplier4/1(In1), multiplier1/1(In1)
  u_dc_link_voltage/1 -> t6/4, t6/3, t6/2, t6/1
  Index/1 -> adder/1

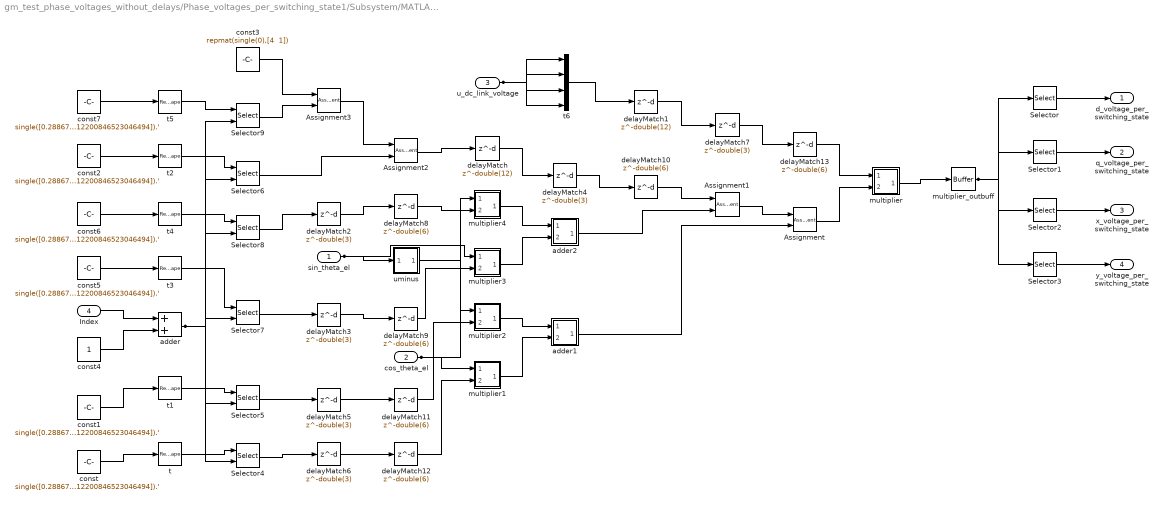
== system gm_test_phase_voltages_without_delays/Phase_voltages_per_switching_state1/Subsystem/MATLAB Function13 ==
  sin_theta_el : Inport  OutDataTypeStr=single  PortDimensions=1  SampleTime=1e-08
  cos_theta_el : Inport  Port=2  OutDataTypeStr=single  PortDimensions=1  SampleTime=1e-08
  u_dc_link_voltage : Inport  Port=3  OutDataTypeStr=single  PortDimensions=1  SampleTime=1e-08
  Index : Inport  Port=4  OutDataTypeStr=int32  PortDimensions=1  SampleTime=1e-08
  Assignment : Assignment  NumberOfDimensions=2  SampleTime=1e-08  IndexOptions=Index vector (dialog),Index vector (dialog)  Indices=double(2),double(1)  OutputSizes=double(0),double(0)
  Assignment1 : Assignment  NumberOfDimensions=2  SampleTime=1e-08  IndexOptions=Index vector (dialog),Index vector (dialog)  Indices=double(1),double(1)  OutputSizes=double(0),double(0)
  Assignment2 : Assignment  NumberOfDimensions=2  SampleTime=1e-08  IndexOptions=Index vector (dialog),Index vector (dialog)  Indices=double(4),double(1)  OutputSizes=double(0),double(0)
  Assignment3 : Assignment  NumberOfDimensions=2  SampleTime=1e-08  IndexOptions=Index vector (dialog),Index vector (dialog)  Indices=double(3),double(1)  OutputSizes=double(0),double(0)
  Selector : Selector  NumberOfDimensions=2  SampleTime=1e-08  IndexOptions=Index vector (dialog),Index vector (dialog)  Indices=double(1),double(1)  OutputSizes=double(0),double(0)
  Selector1 : Selector  NumberOfDimensions=2  SampleTime=1e-08  IndexOptions=Index vector (dialog),Index vector (dialog)  Indices=double(2),double(1)  OutputSizes=double(0),double(0)
  Selector2 : Selector  NumberOfDimensions=2  SampleTime=1e-08  IndexOptions=Index vector (dialog),Index vector (dialog)  Indices=double(3),double(1)  OutputSizes=double(0),double(0)
  Selector3 : Selector  NumberOfDimensions=2  SampleTime=1e-08  IndexOptions=Index vector (dialog),Index vector (dialog)  Indices=double(4),double(1)  OutputSizes=double(0),double(0)
  Selector4 : Selector  NumberOfDimensions=2  SampleTime=1e-08  IndexOptions=Index vector (dialog),Index vector (port)  Indices=double(2),double(-1)  OutputSizes=double(0),double(0)
  Selector5 : Selector  NumberOfDimensions=2  SampleTime=1e-08  IndexOptions=Index vector (dialog),Index vector (port)  Indices=double(1),double(-1)  OutputSizes=double(0),double(0)
  Selector6 : Selector  NumberOfDimensions=2  SampleTime=1e-08  IndexOptions=Index vector (dialog),Index vector (port)  Indices=double(4),double(-1)  OutputSizes=double(0),double(0)
  Selector7 : Selector  NumberOfDimensions=2  SampleTime=1e-08  IndexOptions=Index vector (dialog),Index vector (port)  Indices=double(2),double(-1)  OutputSizes=double(0),double(0)
  Selector8 : Selector  NumberOfDimensions=2  SampleTime=1e-08  IndexOptions=Index vector (dialog),Index vector (port)  Indices=double(1),double(-1)  OutputSizes=double(0),double(0)
  Selector9 : Selector  NumberOfDimensions=2  SampleTime=1e-08  IndexOptions=Index vector (dialog),Index vector (port)  Indices=double(3),double(-1)  OutputSizes=double(0),double(0)
  adder : Sum  AccumDataTypeStr=int32  OutDataTypeStr=int32  RndMeth=Nearest  SaturateOnIntegerOverflow=on  SampleTime=1e-08
  adder1 : Subsystem
      mask Display: disp('NFP\nadd');
  adder2 : Subsystem
      mask Display: disp('NFP\nadd');
  const{,1..2,5..7} (6 alike) : Constant  Value=single([0.28867512941360474 0.1666666716337204 -0.28867512941360474 0.1666666716337204 0.6220084428787231 0.1666666716337204 0.044658198952674866 0.1666666716337204 0.12200846523046494 0.45534181594848633 -0.45534181594848633 -0.12200846523046494 0.45534181594848633 0.45534181594848633 -0.12200846523046494 -0.12200846523046494]).'  VectorParams1D=off  OutDataTypeStr=single  SampleTime=1e-08
  const3 : Constant  Value="repmat(single(0),[4  1])"  VectorParams1D=off  OutDataTypeStr=single  SampleTime=1e-08
  const4 : Constant  VectorParams1D=off  OutDataTypeStr=int32  SampleTime=1e-08
  delayMatch : Delay  DelayLength=double(12)  InitialCondition=0  SampleTime=1e-08
  delayMatch1 : Delay  DelayLength=double(12)  InitialCondition=0  SampleTime=1e-08
  delayMatch{8..13} (6 alike) : Delay  DelayLength=double(6)  InitialCondition=0  SampleTime=1e-08
  delayMatch{2..7} (6 alike) : Delay  DelayLength=double(3)  InitialCondition=0  SampleTime=1e-08
  multiplier : Subsystem
      mask Display: disp('NFP\nmul');
  multiplier1 : Subsystem
      mask Display: disp('NFP\nmul');
  multiplier2 : Subsystem
      mask Display: disp('NFP\nmul');
  multiplier3 : Subsystem
      mask Display: disp('NFP\nmul');
  multiplier4 : Subsystem
      mask Display: disp('NFP\nmul');
  multiplier_outbuff : hdlmdlgenlib/Buffer
      settings: SourceProductBaseCode=SL
  t{,1..5} (6 alike) : Reshape  OutputDimensionality=Customize  OutputDimensions=[4,4]
  t6 : Mux
  uminus : Subsystem
      mask Display: disp('NFP\numinus');
  d_voltage_per_switching_state : Outport  SampleTime=1e-08  VectorParamsAs1DForOutWhenUnconnected=off
  q_voltage_per_switching_state : Outport  Port=2  SampleTime=1e-08
  x_voltage_per_switching_state : Outport  Port=3  SampleTime=1e-08
  y_voltage_per_switching_state : Outport  Port=4  SampleTime=1e-08
  wires:
  Selector/1 -> d_voltage_per_switching_state/1
  Selector1/1 -> q_voltage_per_switching_state/1
  Selector2/1 -> x_voltage_per_switching_state/1
  Selector3/1 -> y_voltage_per_switching_state/1
  multiplier_outbuff/1 -> Selector3/1, Selector2/1, Selector1/1, Selector/1
  Assignment/1 -> multiplier/2(In2)
  Assignment1/1 -> Assignment/1
  delayMatch10/1 -> Assignment1/1
  delayMatch12/1 -> multiplier1/2(In2)
  delayMatch11/1 -> multiplier2/2(In2)
  Selector6/1 -> Assignment2/2
  Assignment3/1 -> Assignment2/1
  adder/1 -> Selector9/2, Selector8/2, Selector7/2, Selector6/2, Selector5/2, Selector4/2
  t/1 -> Selector4/1
  t1/1 -> Selector5/1
  delayMatch9/1 -> multiplier3/2(In2)
  delayMatch8/1 -> multiplier4/2(In2)
  t2/1 -> Selector6/1
  Selector9/1 -> Assignment3/2
  const3/1 -> Assignment3/1
  const4/1 -> adder/2
  t3/1 -> Selector7/1
  t4/1 -> Selector8/1
  t5/1 -> Selector9/1
  const/1 -> t/1
  const1/1 -> t1/1
  const2/1 -> t2/1
  const5/1 -> t3/1
  const6/1 -> t4/1
  const7/1 -> t5/1
  delayMatch13/1 -> multiplier/1(In1)
  multiplier/1(Out1) -> multiplier_outbuff/1
  adder1/1(Out1) -> Assignment/2
  multiplier1/1(Out1) -> adder1/2(In2)
  multiplier2/1(Out1) -> adder1/1(In1)
  adder2/1(Out1) -> Assignment1/2
  uminus/1(Out1) -> multiplier2/1(In1)
  multiplier3/1(Out1) -> adder2/2(In2)
  multiplier4/1(Out1) -> adder2/1(In1)
  Assignment2/1 -> delayMatch/1
  t6/1 -> delayMatch1/1
  Selector8/1 -> delayMatch2/1
  Selector7/1 -> delayMatch3/1
  delayMatch/1 -> delayMatch4/1
  Selector5/1 -> delayMatch5/1
  Selector4/1 -> delayMatch6/1
  delayMatch1/1 -> delayMatch7/1
  delayMatch2/1 -> delayMatch8/1
  delayMatch3/1 -> delayMatch9/1
  delayMatch4/1 -> delayMatch10/1
  delayMatch5/1 -> delayMatch11/1
  delayMatch6/1 -> delayMatch12/1
  delayMatch7/1 -> delayMatch13/1
  sin_theta_el/1 -> multiplier3/1(In1), uminus/1(In1)
  cos_theta_el/1 -> multiplier4/1(In1), multiplier1/1(In1)
  u_dc_link_voltage/1 -> t6/4, t6/3, t6/2, t6/1
  Index/1 -> adder/1
